simulink model "gm_bit_mapping_model"  (R2020b)
settings: Solver=FixedStepDiscrete  StartTime=0.0  StopTime=30  RelTol=1e-3
libraries: hdlmdlgenlib x2, commrandsrc3 x1
settings Model: Creator=wardo  LastModifiedBy=wardo
settings OptimizationCC: BlockReduction=off  ConditionallyExecuteInputs=off  DefaultParameterBehavior=Inlined
settings DebuggingCC: AlgebraicLoopMsg=error  InheritedTsInSrcMsg=none  SingleTaskRateTransMsg=error
settings HardwareCC: ProdBitPerPointer=32  ProdBitPerSizeT=32  ProdBitPerPtrDiffT=32  ProdLargestAtomicFloat=None  ProdIntDivRoundTo=Undefined  ProdEndianess=Unspecified  ProdWordSize=32  ProdHWDeviceType=ASIC/FPGA->ASIC/FPGA  TargetBitPerLong=64  TargetBitPerPointer=64  TargetBitPerSizeT=64  TargetBitPerPtrDiffT=64  TargetLongLongMode=on  TargetIntDivRoundTo=Zero  TargetEndianess=LittleEndian  TargetWordSize=64  TargetHWDeviceType=Custom Processor->MATLAB Host Computer  ProdEqTarget=off

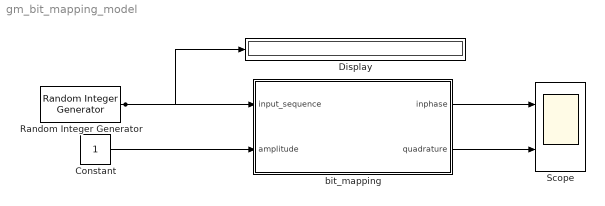
== system gm_bit_mapping_model ==
  Constant : Constant  OutMin=0  OutMax=5  OutDataTypeStr=fixdt(1,16)  SampleTime=-1
  Display : Display
  Random Integer Generator : commrandsrc3/Random Integer Generator  SetSize=2  SeedSource=Auto  Seed=0  SampleTime=1  SamplesPerFrame=3  OutputDataType=boolean  SimulateUsing=Interpreted execution
  Scope : Scope  NumInputPorts=2
  bit_mapping : Subsystem
  wires:
  bit_mapping/1(inphase) -> Scope/1
  Random Integer Generator/1 -> bit_mapping/1(input_sequence), Display/1
  Constant/1 -> bit_mapping/2(amplitude)
  bit_mapping/2(quadrature) -> Scope/2

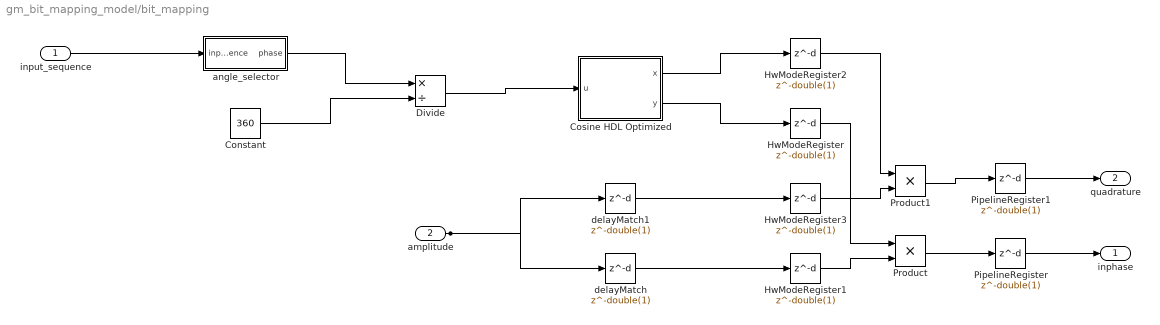
== system gm_bit_mapping_model/bit_mapping ==
  input_sequence : Inport  OutDataTypeStr=boolean  PortDimensions=[3 1]  SampleTime=3
  amplitude : Inport  Port=2  OutDataTypeStr=fixdt(1, 16, 12)  PortDimensions=1  SampleTime=3
  Constant : Constant  Value=360  OutDataTypeStr=fixdt(0, 9, 0)  SampleTime=3
  Cosine HDL Optimized : Subsystem  mask(Sine and Cosine HDL optimized block){OutputFormula=sin(2*pi*u) and cos(2*pi*u), NumDataPoints=double(32), TableDataTypeStr=fixdt(1,16,15), SimulateLUTROMDelay=off}
      mask prompts: OutputFormula "Simulink:masks:OutputFormula_MP"; NumDataPoints "HDLShared:hdlshared:CosineHDL_Npts"; TableDataTypeStr "Simulink:blkprm_prompts:TABLE_UNIFIEDDATATYPE"; SimulateLUTROMDelay "HDLShared:hdlshared:CosineHDL_Map2RAM"
      mask help: Sine and Cosine HDL optimized block using quarter wave symmetry, and HDL friendly settings.
      mask Help: helpview([docroot '/hdlcoder/helptargets.map'],'SineAndCosineHDL_Optimized');
      mask TypeOptions OutputFormula: sin(2*pi*u) | cos(2*pi*u) | exp(j*2*pi*u) | sin(2*pi*u) and cos(2*pi*u)
      mask Display:
      | port_label('input',1,'u')
      | port_label('output',1,'sin(2*pi*u)')
      | port_label('output',2,'cos(2*pi*u)')
      | xpos = 0.35;
      | yoffset = 0.5;
      | if ( SimulateLUTROMDelay )
      |   text(xpos,yoffset,'HDL (Z^{-1})','texmode','on')
      | else
      |    text(xpos,yoffset,'HDL')
      | end
  Divide : Product  Inputs=*/  OutDataTypeStr=fixdt(1, 16, 14)  RndMeth=Zero  SaturateOnIntegerOverflow=on  SampleTime=3
  HwModeRegister{,1..3} (4 alike) : Delay  DelayLength=double(1)  InitialCondition=0  SampleTime=3
  PipelineRegister : Delay  DelayLength=double(1)  InitialCondition=0  SampleTime=3
  PipelineRegister1 : Delay  DelayLength=double(1)  InitialCondition=0  SampleTime=3
  Product : Product  Inputs=**  OutDataTypeStr=fixdt(1, 33, 27)  SampleTime=3
  Product1 : Product  Inputs=**  OutDataTypeStr=fixdt(1, 33, 27)  SampleTime=3
  angle_selector : Subsystem
  delayMatch : Delay  DelayLength=double(1)  InitialCondition=0  SampleTime=3
  delayMatch1 : Delay  DelayLength=double(1)  InitialCondition=0  SampleTime=3
  inphase : Outport  VectorParamsAs1DForOutWhenUnconnected=off
  quadrature : Outport  Port=2  VectorParamsAs1DForOutWhenUnconnected=off
  wires:
  input_sequence/1 -> angle_selector/1(input_sequence)
  delayMatch/1 -> HwModeRegister1/1
  Constant/1 -> Divide/2
  Cosine HDL Optimized/1(x) -> HwModeRegister2/1
  Cosine HDL Optimized/2(y) -> HwModeRegister/1
  Divide/1 -> Cosine HDL Optimized/1(u)
  PipelineRegister/1 -> inphase/1
  PipelineRegister1/1 -> quadrature/1
  angle_selector/1(phase) -> Divide/1
  delayMatch1/1 -> HwModeRegister3/1
  amplitude/1 -> delayMatch1/1, delayMatch/1
  Product/1 -> PipelineRegister/1
  HwModeRegister/1 -> Product/1
  HwModeRegister1/1 -> Product/2
  Product1/1 -> PipelineRegister1/1
  HwModeRegister2/1 -> Product1/1
  HwModeRegister3/1 -> Product1/2

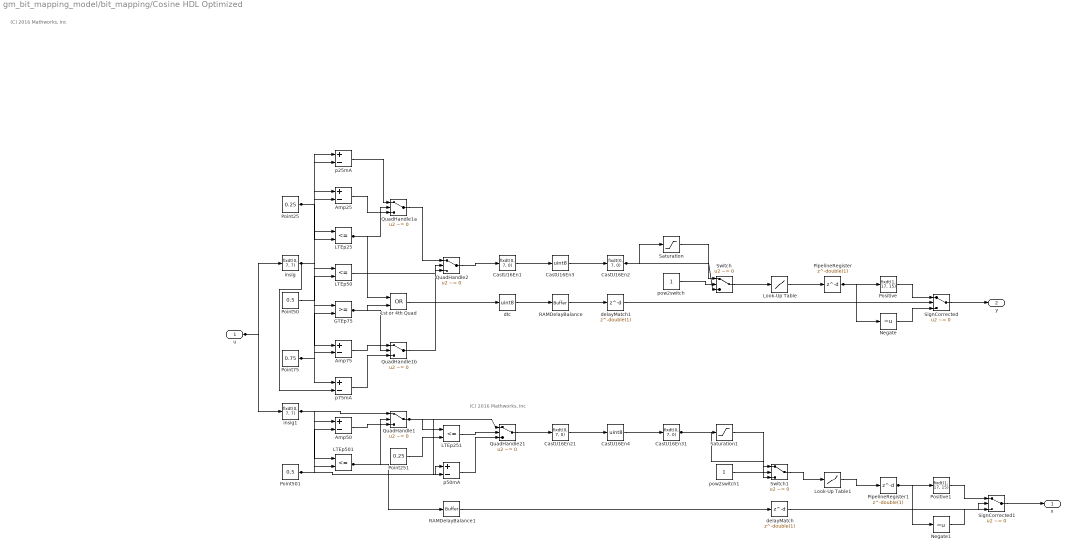
== system gm_bit_mapping_model/bit_mapping/Cosine HDL Optimized ==
  note: (C) 2016 Mathworks, Inc
  note: (C) 2016 Mathworks, Inc
  u : Inport  OutDataTypeStr=fixdt(1, 16, 14)  SampleTime=3
  1st or 4th Quad : Logic  Operator=OR  AllPortsSameDT=off  OutDataTypeStr=boolean  SampleTime=3
  Amp25 : Sum  Inputs=+-  AccumDataTypeStr=fixdt(1, 18, 17)  OutDataTypeStr=fixdt(1, 18, 17)  SampleTime=3
  Amp50 : Sum  Inputs=+-  AccumDataTypeStr=fixdt(1, 18, 17)  OutDataTypeStr=fixdt(1, 18, 17)  SampleTime=3
  Amp75 : Sum  Inputs=+-  AccumDataTypeStr=fixdt(1, 18, 17)  OutDataTypeStr=fixdt(1, 18, 17)  SampleTime=3
  CastU16En1 : DataTypeConversion  OutDataTypeStr=fixdt(0, 7, 0)  ConvertRealWorld=Stored Integer (SI)  SampleTime=3
  CastU16En2 : DataTypeConversion  OutDataTypeStr=fixdt(0, 7, 0)  ConvertRealWorld=Stored Integer (SI)  SampleTime=3  SaturateOnIntegerOverflow=on
  CastU16En21 : DataTypeConversion  OutDataTypeStr=fixdt(0, 7, 0)  ConvertRealWorld=Stored Integer (SI)  SampleTime=3
  CastU16En3 : DataTypeConversion  OutDataTypeStr=uint8  SampleTime=3
  CastU16En31 : DataTypeConversion  OutDataTypeStr=fixdt(0, 7, 0)  ConvertRealWorld=Stored Integer (SI)  SampleTime=3  SaturateOnIntegerOverflow=on
  CastU16En4 : DataTypeConversion  OutDataTypeStr=uint8  SampleTime=3
  GTEp75 : RelationalOperator  OutDataTypeStr=boolean  SampleTime=3  RndMeth=Nearest
  LTEp{25,50,251,501} (4 alike) : RelationalOperator  Operator=<=  OutDataTypeStr=boolean  SampleTime=3  RndMeth=Nearest
  Look-Up Table : Lookup_n-D  NumberOfTableDimensions=1  BreakpointsForDimension1="fi(\"numerictype\",numerictype(0,7,0),\"fimath\",fimath(\"RoundingMethod\", \"Floor\",\"OverflowAction\", \"Wrap\",\"ProductMode\",\"FullPrecision\",\"SumMode\",\"FullPrecision\"),\"Value\",\"[0 1 2 3 4 5 6 7 8 9 10 11 12 13 14 15 16 17 18 19 20 21 22 23 24 25 26 27 28 29 30 31]\")"  Table="reshape(fi(\"numerictype\",numerictype(1,17,15),\"fimath\",fimath(\"RoundingMethod\", \"Floor\",\"OverflowAction\", \"Wrap\",\"ProductMode\",\"FullPrecision\",\"SumMode\",\"FullPrecision\"),\"Value\",\"[0;0.0506591796875;0.101165771484375;0.15142822265625;0.2012939453125;0.250640869140625;0.29937744140625;0.3472900390625;0.39434814453125;0.440399169921875;0.48529052734375;0.528961181640625;0.571258544921875;0.612091064453125;0.6513671875;0.68896484375;0.72479248046875;0.758758544921875;0.790771484375;0.820770263671875;0.8486328125;0.874359130859375;0.897796630859375;0.9189453125;0.937744140625;0.954132080078125;0.96807861328125;0.979522705078125;0.98846435546875;0.994873046875;0.99871826171875;1]\"), [1  32])"  InterpMethod=Flat  ExtrapMethod=Clip  DiagnosticForOutOfRangeInput=Error  SampleTime=3  OutDataTypeStr=fixdt(1, 17, 15)  InputSameDT=on
  Look-Up Table1 : Lookup_n-D  NumberOfTableDimensions=1  BreakpointsForDimension1="fi(\"numerictype\",numerictype(0,7,0),\"fimath\",fimath(\"RoundingMethod\", \"Floor\",\"OverflowAction\", \"Wrap\",\"ProductMode\",\"FullPrecision\",\"SumMode\",\"FullPrecision\"),\"Value\",\"[0 1 2 3 4 5 6 7 8 9 10 11 12 13 14 15 16 17 18 19 20 21 22 23 24 25 26 27 28 29 30 31]\")"  Table="reshape(fi(\"numerictype\",numerictype(1,17,15),\"fimath\",fimath(\"RoundingMethod\", \"Floor\",\"OverflowAction\", \"Wrap\",\"ProductMode\",\"FullPrecision\",\"SumMode\",\"FullPrecision\"),\"Value\",\"[0;0.0506591796875;0.101165771484375;0.15142822265625;0.2012939453125;0.250640869140625;0.29937744140625;0.3472900390625;0.39434814453125;0.440399169921875;0.48529052734375;0.528961181640625;0.571258544921875;0.612091064453125;0.6513671875;0.68896484375;0.72479248046875;0.758758544921875;0.790771484375;0.820770263671875;0.8486328125;0.874359130859375;0.897796630859375;0.9189453125;0.937744140625;0.954132080078125;0.96807861328125;0.979522705078125;0.98846435546875;0.994873046875;0.99871826171875;1]\"), [1  32])"  InterpMethod=Flat  ExtrapMethod=Clip  DiagnosticForOutOfRangeInput=Error  SampleTime=3  OutDataTypeStr=fixdt(1, 17, 15)  InputSameDT=on
  Negate : UnaryMinus  SampleTime=3
  Negate1 : UnaryMinus  SampleTime=3
  PipelineRegister : Delay  DelayLength=double(1)  InitialCondition=0  SampleTime=3
  PipelineRegister1 : Delay  DelayLength=double(1)  InitialCondition=0  SampleTime=3
  Point25 : Constant  Value=0.25  OutDataTypeStr=fixdt(0, 17, 17)  SampleTime=3
  Point251 : Constant  Value=0.25  OutDataTypeStr=fixdt(0, 17, 17)  SampleTime=3
  Point50 : Constant  Value=0.5  OutDataTypeStr=fixdt(0, 17, 17)  SampleTime=3
  Point501 : Constant  Value=0.5  OutDataTypeStr=fixdt(0, 17, 17)  SampleTime=3
  Point75 : Constant  Value=0.75  OutDataTypeStr=fixdt(0, 17, 17)  SampleTime=3
  Positive : DataTypeConversion  OutDataTypeStr=fixdt(1, 17, 15)  SampleTime=3
  Positive1 : DataTypeConversion  OutDataTypeStr=fixdt(1, 17, 15)  SampleTime=3
  QuadHandle1 : Switch  Criteria=u2 ~= 0  Threshold=double(0)  OutDataTypeStr=fixdt(1, 18, 17)  SampleTime=3
  QuadHandle1a : Switch  Criteria=u2 ~= 0  Threshold=double(0)  OutDataTypeStr=fixdt(1, 18, 17)  SampleTime=3
  QuadHandle1b : Switch  Criteria=u2 ~= 0  Threshold=double(0)  OutDataTypeStr=fixdt(1, 18, 17)  SampleTime=3
  QuadHandle2 : Switch  Criteria=u2 ~= 0  Threshold=double(0)  OutDataTypeStr=fixdt(0, 7, 7)  SampleTime=3  SaturateOnIntegerOverflow=on
  QuadHandle21 : Switch  Criteria=u2 ~= 0  Threshold=double(0)  OutDataTypeStr=fixdt(0, 7, 7)  SampleTime=3
  RAMDelayBalance : hdlmdlgenlib/Buffer
      settings: SourceProductBaseCode=SL
  RAMDelayBalance1 : hdlmdlgenlib/Buffer
      settings: SourceProductBaseCode=SL
  Saturation : Saturate  UpperLimit="fi(0,0,7,0,\"hex\",\"1f\")"  LowerLimit="fi(0,0,7,0,\"hex\",\"00\")"  SampleTime=3  OutDataTypeStr=fixdt(0, 7, 0)
  Saturation1 : Saturate  UpperLimit="fi(0,0,7,0,\"hex\",\"1f\")"  LowerLimit="fi(0,0,7,0,\"hex\",\"00\")"  SampleTime=3  OutDataTypeStr=fixdt(0, 7, 0)
  SignCorrected : Switch  Criteria=u2 ~= 0  Threshold=double(0)  OutDataTypeStr=fixdt(1, 17, 15)  SampleTime=3
  SignCorrected1 : Switch  Criteria=u2 ~= 0  Threshold=double(0)  OutDataTypeStr=fixdt(1, 17, 15)  SampleTime=3
  Switch : Switch  Criteria=u2 ~= 0  Threshold=double(0)  OutDataTypeStr=fixdt(0, 7, 0)  SampleTime=3
  Switch1 : Switch  Criteria=u2 ~= 0  Threshold=double(0)  OutDataTypeStr=fixdt(0, 7, 0)  SampleTime=3
  delayMatch : Delay  DelayLength=double(1)  InitialCondition=0  SampleTime=3
  delayMatch1 : Delay  DelayLength=double(1)  InitialCondition=0  SampleTime=3
  dtc : DataTypeConversion  OutDataTypeStr=uint8  SampleTime=3
  insig : DataTypeConversion  OutDataTypeStr=fixdt(0, 7, 7)  SampleTime=3
  insig1 : DataTypeConversion  OutDataTypeStr=fixdt(0, 7, 7)  SampleTime=3
  p25mA : Sum  Inputs=+-  AccumDataTypeStr=fixdt(1, 18, 17)  OutDataTypeStr=fixdt(1, 18, 17)  SampleTime=3
  p50mA : Sum  Inputs=+-  AccumDataTypeStr=fixdt(1, 19, 17)  OutDataTypeStr=fixdt(1, 19, 17)  SampleTime=3
  p75mA : Sum  Inputs=+-  AccumDataTypeStr=fixdt(1, 18, 17)  OutDataTypeStr=fixdt(1, 18, 17)  SampleTime=3
  pow2switch : Constant  OutDataTypeStr=boolean  SampleTime=3
  pow2switch1 : Constant  OutDataTypeStr=boolean  SampleTime=3
  x : Outport
  y : Outport  Port=2
  wires:
  dtc/1 -> RAMDelayBalance/1
  Amp25/1 -> QuadHandle1a/3
  Amp75/1 -> QuadHandle1b/1
  CastU16En1/1 -> CastU16En3/1
  CastU16En2/1 -> Switch/3, Saturation/1
  CastU16En3/1 -> CastU16En2/1
  GTEp75/1 -> QuadHandle1b/2, 1st or 4th Quad/2
  LTEp25/1 -> QuadHandle1a/2, 1st or 4th Quad/1
  LTEp50/1 -> QuadHandle2/2
  PipelineRegister/1 -> Positive/1, Negate/1
  Negate/1 -> SignCorrected/3
  Point25/1 -> p25mA/1, LTEp25/2, Amp25/2
  Point50/1 -> LTEp50/2
  Point75/1 -> p75mA/1, GTEp75/2, Amp75/2
  Positive/1 -> SignCorrected/1
  QuadHandle1a/1 -> QuadHandle2/1
  QuadHandle1b/1 -> QuadHandle2/3
  QuadHandle2/1 -> CastU16En1/1
  delayMatch1/1 -> SignCorrected/2
  Saturation/1 -> Switch/1
  SignCorrected/1 -> y/1
  Switch/1 -> Look-Up Table/1
  insig/1 -> p75mA/2, p25mA/2, LTEp50/1, LTEp25/1, GTEp75/1, Amp75/1, Amp25/1
  p25mA/1 -> QuadHandle1a/1
  p75mA/1 -> QuadHandle1b/3
  pow2switch/1 -> Switch/2
  Amp50/1 -> QuadHandle1/3
  CastU16En21/1 -> CastU16En4/1
  CastU16En31/1 -> Switch1/3, Saturation1/1
  CastU16En4/1 -> CastU16En31/1
  LTEp251/1 -> QuadHandle21/2
  LTEp501/1 -> QuadHandle1/2, RAMDelayBalance1/1
  PipelineRegister1/1 -> Positive1/1, Negate1/1
  Negate1/1 -> SignCorrected1/3
  Point251/1 -> LTEp251/2
  Point501/1 -> p50mA/1, LTEp501/2, Amp50/2
  Positive1/1 -> SignCorrected1/1
  QuadHandle1/1 -> p50mA/2, QuadHandle21/1, LTEp251/1
  QuadHandle21/1 -> CastU16En21/1
  delayMatch/1 -> SignCorrected1/2
  Saturation1/1 -> Switch1/1
  SignCorrected1/1 -> x/1
  Switch1/1 -> Look-Up Table1/1
  insig1/1 -> QuadHandle1/1, LTEp501/1, Amp50/1
  p50mA/1 -> QuadHandle21/3
  pow2switch1/1 -> Switch1/2
  1st or 4th Quad/1 -> dtc/1
  RAMDelayBalance1/1 -> delayMatch/1
  RAMDelayBalance/1 -> delayMatch1/1
  u/1 -> insig1/1, insig/1
  Look-Up Table/1 -> PipelineRegister/1
  Look-Up Table1/1 -> PipelineRegister1/1

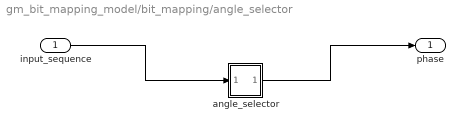
== system gm_bit_mapping_model/bit_mapping/angle_selector ==
  input_sequence : Inport  OutDataTypeStr=boolean  PortDimensions=[3 1]  SampleTime=3
  angle_selector : MATLAB Function  TreatAsAtomicUnit=on
  phase : Outport  VectorParamsAs1DForOutWhenUnconnected=off
  wires:
  angle_selector/1(phase) -> phase/1
  input_sequence/1 -> angle_selector/1(input_sequence)

== matlab function gm_bit_mapping_model/bit_mapping/angle_selector/angle_selector ==
  settings: fimath=fimath('RoundingMethod', 'Floor','OverflowAction', 'Wrap','ProductMode', 'FullPrecision', 'SumMode', 'FullPrecision')
  data: input_sequence input; phase output
function phase = phase_selector(input_sequence)
%#codegen
% Receives a bit sequence and returns the angle in radians of the
% corresponding 8-psk constellation symbol. Gray encoding is used as stated
% in the DVB-S2 standard.
    tmp = 0; % Start at phase 0
    if(input_sequence(1)==0 && input_sequence(2)==0 && input_sequence(3)==1)
        tmp=0;
    elseif(input_sequence(1)==0 && input_sequence(2)==0 && input_sequence(3)==0)
        tmp=45;
    elseif(input_sequence(1)==1 && input_sequence(2)==0 && input_sequence(3)==0)
        tmp=90;
    elseif(input_sequence(1)==1 && input_sequence(2)==1 && input_sequence(3)==0)
        tmp=135;
    elseif(input_sequence(1)==0 && input_sequence(2)==1 && input_sequence(3)==0)
        tmp=180;
    elseif(input_sequence(1)==0 && input_sequence(2)==1 && input_sequence(3)==1)
        tmp=225;
    elseif(input_sequence(1)==1 && input_sequence(2)==1 && input_sequence(3)==1)
        tmp=270;
    elseif(input_sequence(1)==1 && input_sequence(2)==0 && input_sequence(3)==1)
        tmp=315;
    end
    % 9 bits necessary to represent 360 degrees.
    phase = fi(tmp, 0, 23, 14, hdlfimath);
